simulink model "MotoSim"  (Simulink 8.9)
settings: Solver=ode1  StartTime=0.0  StopTime=Inf  FixedStep=0.01  RelTol=1e-3  EnableMultiTasking=on
PreLoadFcn:
  | clear all
  | close all
  | clc
  | 
  | currentFolder = pwd;
  | addpath(genpath(currentFolder));
values from neighbouring files (symbols this model uses):
  Stoptime = 60    [Initialize_Environment.m]    (also in Initialize_Environment_CDTS.m; Initialize_Environment_combined.m; Initialize_Sim.m)
undefined symbols (not defined in the file or in its folder): BATT_ELEC, BATT_OCV, BATT_THERMAL, EM, MC, soc0
libraries: simulink x4
settings Model: Creator=bring  LastModifiedBy=bring
settings OptimizationCC: ExpressionDepthLimit=2147483647
settings DebuggingCC: CheckSSInitialOutputMsg=off  SolverPrmCheckMsg=warning
settings SFSimCC: SimParseCustomCode=off
settings ConfigComp: CovSFcnEnable=off

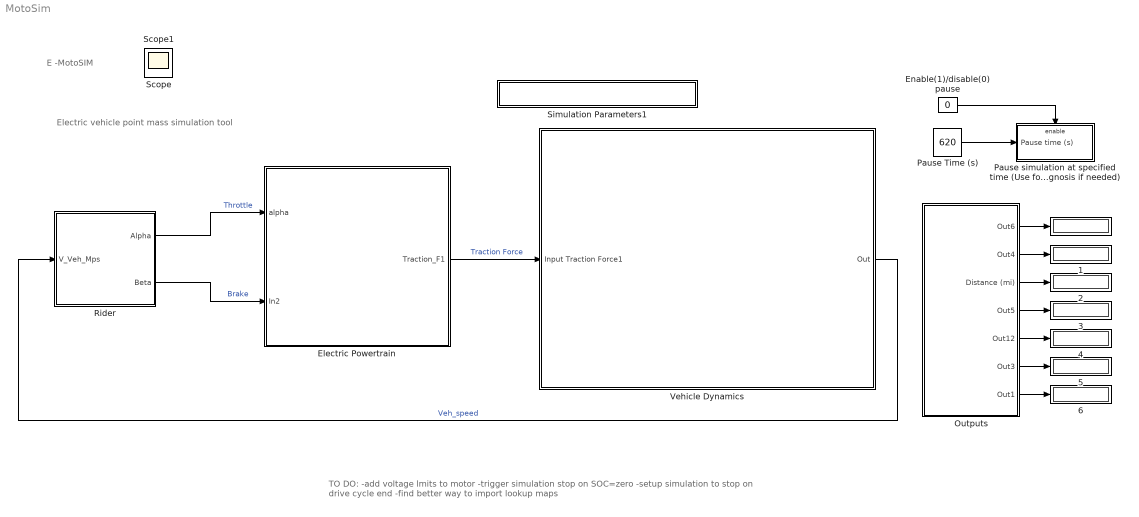
== system MotoSim ==
  note: TO DO:
      | -add voltage lmits to motor
      | -trigger simulation stop on SOC=zero
      | -setup simulation to stop on drive cycle end
      | -find better way to import lookup maps
  note: Electric vehicle point mass simulation tool
  note: E -MotoSIM
   {,1..6} (7 alike) : Display
  Electric Powertrain : Subsystem
      mask Display: image(imread('images/bike_powertrain.jpg'))
  Enable(1)/disable(0) pause : Constant  Value=0
  Outputs : Subsystem  mask(Outputs){}
  Pause Time (s) : Constant  Value=620
  Pause simulation at specified time (Use for diagnosis if needed) : Subsystem
  Rider : Subsystem  mask(Driver){kp=1, ki=0.1, kd=0.1}
      mask prompts: kp "Proportional Gain"; ki "Integral Gain"; kd "Derivative Gain"
      mask help: Please select the PID controller gains to improve the tracking response.
      mask Display: image(imread('Images/helmet.jpg'))
  Simulation Parameters1 : Subsystem  mask(Simulation Options){DRIV_Cycle=FUDS, VEH_Selection=sportbike_generic, M=250, TIRE_radius=0.3, CdA=0.38, maxBrakeTorque=2000, rowA=1.2, FrontSprocket_toothCt=23, RearSprocket_toothCt=54, regenPct=0, EM_MC_Selection=emrax268_PM150DZR, CELL_Selection=LiFePo4_generic, cellSeriesCount=134, cellParallelCount=1, cellCapacity=20, ENV_Selection=TRC_VDA, ambTemp=20, soc0=90, Grade_Value=0, Wind_Speed=0, iteration=1, DRIV_acc_flag=off, DRIV_acc_final_v=100}
      mask prompts: DRIV_Cycle "Driving Cycle"; VEH_Selection "Vehicle Selection"; M "Vehicle+Rider Mass (kg)"; TIRE_radius "Tire Radius"; maxBrakeTorque "Max Brake Torque"; rowA "Air Density"; FrontSprocket_toothCt "Fr Sprocket Teeth"; RearSprocket_toothCt "Rr Sprocket Teeth"; regenPct "Regen %"; EM_MC_Selection "Motor-MC Selection"; CELL_Selection "Battery Cell Selection"; cellSeriesCount "Series Cells"; cellParallelCount "Parallel Cells"; cellCapacity "Cell Capacity (Ah)"; ENV_Selection "Environment Selection"; ambTemp "Ambient Temperature (C)"; soc0 "Battey Initial SOC (%)"; Grade_Value "Road Grade Climb (degrees)"; Wind_Speed "Wind Speed (m/s)"; iteration "Driving Cycle Repetition"; DRIV_acc_flag "Acceleration Test"; DRIV_acc_final_v "Acceleration Test Final Velocity [kmph]"
      mask TypeOptions DRIV_Cycle: FHDS | FUDS | FUDS_fast | WLTP | US06 | US06_City_Cycle | US06_Highway_Cycle | Artemis_urban | Artemis_extra_urban | Artemis_highway | NEDC | PPIHC_CDTS
      mask TypeOptions VEH_Selection: sportbike_generic | EXR100 | RW-3x
      mask TypeOptions EM_MC_Selection: emrax268_PM150DZR | ME708_KDS48200e
      mask TypeOptions CELL_Selection: LiFePo4_generic | A123_ANR26650
      mask TypeOptions ENV_Selection: TRC_VDA | PikesPeak
      mask Display: text(.5,.5,'\fontsize{10}{\bfSimulation Settings}', 'hor','center','texmode','on');
  Vehicle Dynamics : Subsystem
      mask Display: image(imread('images/bike.jpg'))
  Scope : Scope
  Scope1 : Scope
  wires:
  Vehicle Dynamics/1(Out) -> Rider/1(V_Veh_Mps)  "Veh_speed"
  Rider/2(Beta) -> Electric Powertrain/2(In2)  "Brake"
  Rider/1(Alpha) -> Electric Powertrain/1(alpha)  "Throttle"
  Electric Powertrain/1(Traction_F1) -> Vehicle Dynamics/1(Input Traction Force1)  "Traction Force"
  Pause Time (s)/1 -> Pause simulation at specified time (Use for diagnosis if needed)/1(Pause time (s))
  Enable(1)/disable(0) pause/1 -> Pause simulation at specified time (Use for diagnosis if needed)/Enable
  Outputs/7(Out1) -> " 6"/1
  Outputs/6(Out3) -> " 5"/1
  Outputs/5(Out12) -> " 4"/1
  Outputs/4(Out5) -> " 3"/1
  Outputs/3(Distance (mi)) -> " 2"/1
  Outputs/2(Out4) -> " 1"/1
  Outputs/1(Out6) -> " "/1

== system MotoSim/Electric Powertrain ==
  alpha : Inport
  In2 : Inport  Port=2
  Battery Pack : Subsystem
      mask Display: image(imread('Images/pack.jpg'))
  Electric Motor  and  Motor Controller : Subsystem
      mask Display: image(imread('Images/idu.jpg'))
  Final Drive : Subsystem
      mask Display: image(imread('Images/gear.jpg'))
  Powertrain Controller : Subsystem
  Sum1 : Sum  Inputs=+|+
  Vehicle Brakes Front : Subsystem  mask(Brake){Brake_Position=[0 .14 0.31 0.46 0.76 1], Brake_Torque=[0 90.3 180.95 270.83 4600.4 6100]}
      mask prompts: Brake_Position "Brake Position"; Brake_Torque "Brake Torque"
      mask help:
      | This block calculates the brake torque using a 1D map between Brake position and Brake Torque
      | The inputs are the Brake Position array between 0 and 1 and the respective Brake Torque values.
      mask Display: image(imread('images/motoBrake.jpg'))
  Vehicle Brakes Rear : Subsystem  mask(Brake){Brake_Position=[0 .14 0.31 0.46 0.76 1], Brake_Torque=[0 90.3 180.95 270.83 4600.4 6100]}
      mask prompts: Brake_Position "Brake Position"; Brake_Torque "Brake Torque"
      mask help:
      | This block calculates the brake torque using a 1D map between Brake position and Brake Torque
      | The inputs are the Brake Position array between 0 and 1 and the respective Brake Torque values.
      mask Display: image(imread('images/motoBrake.jpg'))
  Vehicle Front Wheels : Subsystem
      mask Display: image(imread('Images/frTire_pirelli.jpg'))
  Vehicle Rear Wheels : Subsystem
      mask Display: image(imread('Images/rrTire_pirelli.jpg'))
  Traction_F1 : Outport
  wires:
  Vehicle Brakes Front/1(Out1) -> Vehicle Front Wheels/1(In1)
  alpha/1 -> Powertrain Controller/1(alpha)
  Vehicle Brakes Rear/1(Out1) -> Vehicle Rear Wheels/1(In1)
  In2/1 -> Powertrain Controller/2(In2)
  Powertrain Controller/3(Engine_Torque_Request) -> Vehicle Brakes Rear/2(Beta (Braking))
  Powertrain Controller/1(Engine_Torque_Request3) -> Vehicle Brakes Front/1(Beta (Braking))
  Electric Motor  and  Motor Controller/1(ICE_Speed) -> Final Drive/1(Torque EM)
  Final Drive/1(EM Torque) -> Vehicle Brakes Rear/1(Torque_out_REM_gearbox)
  Sum1/1 -> Traction_F1/1  "Traction Force"
  Vehicle Front Wheels/1(Out1) -> Sum1/1  "Front Traction Force"
  Vehicle Rear Wheels/1(Out1) -> Sum1/2  "Rear Traction Force"
  Powertrain Controller/2(Engine_Torque_Request4) -> Electric Motor  and  Motor Controller/1(Torque EM)

== system MotoSim/Outputs ==
  Battery Outputs : Subsystem
  Driver : Subsystem
  REM Outputs : Subsystem
  Vehicle Parameters : Subsystem
  Out6 : Outport
  Out4 : Outport  Port=2
  Distance (mi) : Outport  Port=3
  Out5 : Outport  Port=4
  Out12 : Outport  Port=5
  Out3 : Outport  Port=6
  Out1 : Outport  Port=7
  wires:
  Battery Outputs/3(Out2) -> Distance (mi)/1
  Battery Outputs/1(Out5) -> Out5/1
  REM Outputs/1(Out7) -> Out3/1
  REM Outputs/2(Out8) -> Out1/1
  Vehicle Parameters/1(Distance (mi)) -> Out4/1  "Distance (mi)"
  Vehicle Parameters/2(Out2) -> Out6/1
  Battery Outputs/2(Out1) -> Out12/1

== system MotoSim/Pause simulation at specified time (Use for diagnosis if needed) ==
  Pause time (s) : Inport
  Enable : EnablePort
  Add1 : Sum  Inputs=+-
  Assertion1 : Assertion  AssertionFailFcn=|  StopWhenAssertionFail=off
      | set_param(bdroot,'SimulationCommand','pause'),
      | disp(sprintf('\nSimulation paused.'))
  Clock1 : Clock
  Compare To Zero1 : simulink/Logic and Bit Operations/Compare To Zero  relop=~=  OutDataTypeStr=boolean
  wires:
  Clock1/1 -> Add1/1
  Compare To Zero1/1 -> Assertion1/1
  Add1/1 -> Compare To Zero1/1
  Pause time (s)/1 -> Add1/2

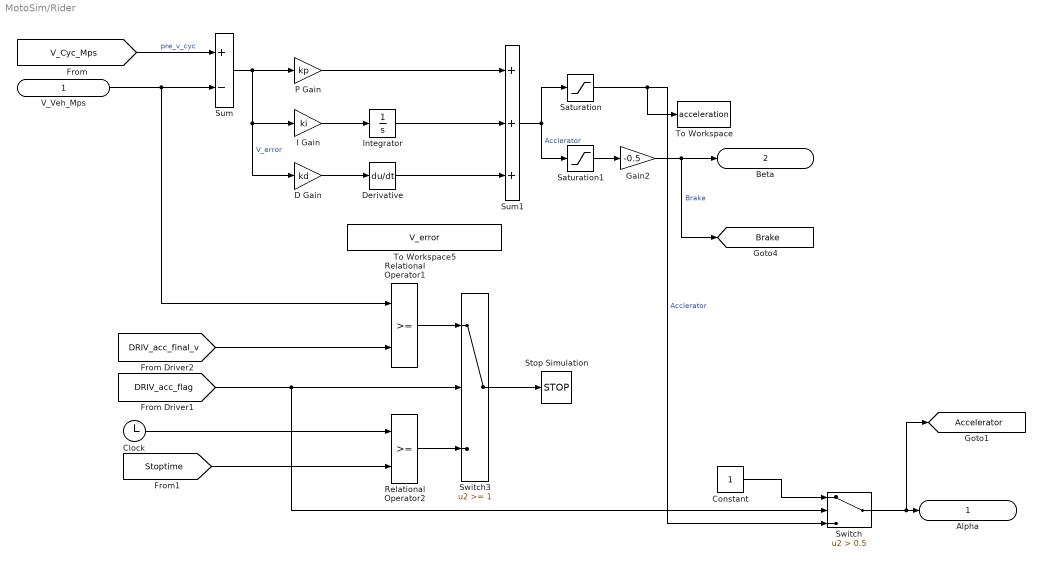
== system MotoSim/Rider ==
  V_Veh_Mps : Inport
  Clock : Clock
  Constant : Constant
  D Gain : Gain  Gain=kd
  Derivative : Derivative
  Gain2 : Gain  Gain=-0.5
  I Gain : Gain  Gain=ki
  Integrator : Integrator  UpperSaturationLimit=0.4
  P Gain : Gain  Gain=kp
  Relational Operator1 : RelationalOperator  RndMeth=Nearest  InputSameDT=on
  Relational Operator2 : RelationalOperator  RndMeth=Nearest  InputSameDT=on
  Saturation : Saturate  UpperLimit=1  LowerLimit=0
  Saturation1 : Saturate  UpperLimit=0  LowerLimit=-1
  Stop Simulation : Stop
  Sum : Sum  Inputs=+-
  Sum1 : Sum  Inputs=+++
  Switch : Switch  Criteria=u2 > Threshold  Threshold=0.5
  Switch3 : Switch  Threshold=1  SaturateOnIntegerOverflow=on  InputSameDT=on
  To Workspace : ToWorkspace  VariableName=acceleration  SampleTime=-1
  To Workspace5 : ToWorkspace  VariableName=V_error  SampleTime=-1
  Alpha : Outport
  Beta : Outport  Port=2
  tag scope: Accelerator=global, Brake=global
  wires:
  Gain2/1 -> [Brake], Beta/1  "Brake"
  Sum1/1 -> Saturation/1, Saturation1/1  "Acclerator"
  D Gain/1 -> Derivative/1
  I Gain/1 -> Integrator/1
  Saturation/1 -> To Workspace/1, Switch/3  "Acclerator"
  Saturation1/1 -> Gain2/1
  Clock/1 -> Relational Operator2/1
  [Stoptime] -> Relational Operator2/2
  [DRIV_acc_flag] -> Switch/2, Switch3/2
  Relational Operator1/1 -> Switch3/1
  [DRIV_acc_final_v] -> Relational Operator1/2
  Switch3/1 -> Stop Simulation/1
  Relational Operator2/1 -> Switch3/3
  Constant/1 -> Switch/1
  Switch/1 -> [Accelerator], Alpha/1
  Derivative/1 -> Sum1/3
  Integrator/1 -> Sum1/2
  P Gain/1 -> Sum1/1
  [V_Cyc_Mps] -> Sum/1  "pre_v_cyc"
  Sum/1 -> P Gain/1, D Gain/1, I Gain/1  "V_error"
  V_Veh_Mps/1 -> Relational Operator1/1, Sum/2

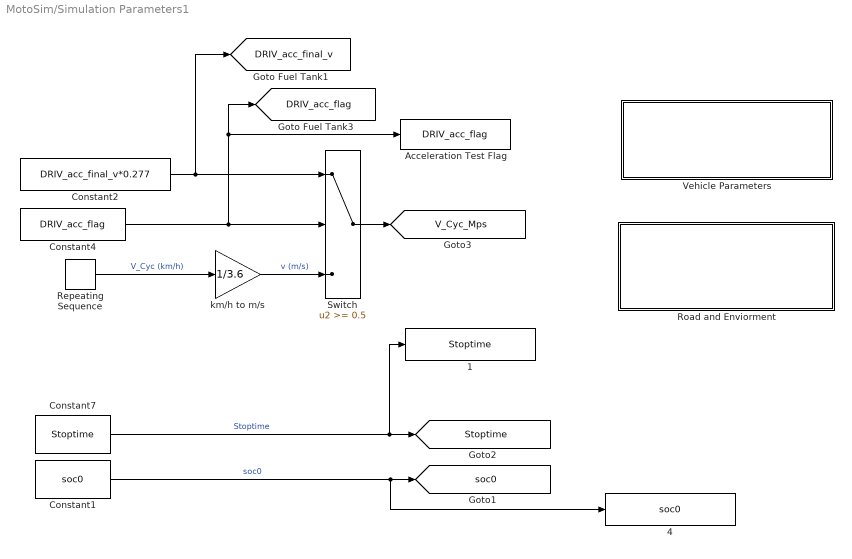
== system MotoSim/Simulation Parameters1 ==
  " 1" : ToWorkspace  VariableName=Stoptime  SampleTime=-1
      settings: MaxDataPoints=1
  " 4" : ToWorkspace  VariableName=soc0  SampleTime=-1
      settings: MaxDataPoints=1
  Acceleration Test Flag : ToWorkspace  VariableName=DRIV_acc_flag  SampleTime=-1
  Constant1 : Constant  Value=soc0
  Constant2 : Constant  Value=DRIV_acc_final_v*0.277
  Constant4 : Constant  Value=DRIV_acc_flag
  Constant7 : Constant  Value=Stoptime
  Repeating Sequence : simulink/Sources/Repeating Sequence  rep_seq_t=t_cyc  rep_seq_y=v_cyc
  Road and Enviorment : Subsystem
      mask Display: text(.5,.5,'\fontsize{10}{ Road and Environment}', 'hor','center','texmode','on');
  Switch : Switch  Threshold=0.5
  Vehicle Parameters : Subsystem
      mask Display: text(.5,.5,'\fontsize{10}{Vehicle Parameters}', 'hor','center','texmode','on');
  km/h to m/s : Gain  Gain=1/3.6
  tag scope: DRIV_acc_final_v=global, DRIV_acc_flag=global, Stoptime=global, V_Cyc_Mps=global, soc0=global
  wires:
  Switch/1 -> [V_Cyc_Mps]
  km/h to m/s/1 -> Switch/3  "v (m/s)"
  Constant2/1 -> Switch/1, [DRIV_acc_final_v]
  Constant4/1 -> Switch/2, [DRIV_acc_flag], Acceleration Test Flag/1
  Constant1/1 -> [soc0], " 4"/1  "soc0"
  Constant7/1 -> [Stoptime], " 1"/1  "Stoptime"
  Repeating Sequence/1 -> km/h to m/s/1  "V_Cyc (km/h)"

== system MotoSim/Vehicle Dynamics ==
  Input Traction Force1 : Inport
  Integrator1 : Integrator
  Saturation : Saturate  UpperLimit=inf  LowerLimit=0
  Vehicle Loads : Subsystem
  Vehicle_speed_Calculation : Subsystem
  Out : Outport
  tag scope: V_at_Wheel=global, Vehicle_Disctance_Travelled=global
  wires:
  Vehicle Loads/1(F (N)) -> Vehicle_speed_Calculation/2(In3)  "Vehicle_load (N)"
  Input Traction Force1/1 -> Vehicle_speed_Calculation/1(In1)
  Vehicle_speed_Calculation/1(Out1) -> Saturation/1  "Vehicle_Speed"
  Integrator1/1 -> [Vehicle_Disctance_Travelled]  "Vehicle_Distance"
  Saturation/1 -> Out/1, [V_at_Wheel], Integrator1/1  "Vehicle_Speed"

== system MotoSim/Electric Powertrain/Battery Pack ==
  Battery Parameters  Calculation : Subsystem
      mask Display:
      | color('blue');
      | fprintf('Battery Parameters Calculation')
  Battery to Cell : Subsystem
      mask Display:
      | color('blue');
      | fprintf('Battery to Cell')
  Cell : Subsystem
      mask Display:
      | color('blue');
      | fprintf('Cell: 1st Order Electrical Model')
  Cell to Batt : Subsystem
      mask Display:
      | color('blue');
      | fprintf('Cell to Battery')
  Current Limiter : Saturate  UpperLimit=180  LowerLimit=-60
  Divide : Product  Inputs=/*
  Memory : Memory
  Sum : Sum
  Thermal Dynamics : Subsystem
      mask Display:
      | color('blue');
      | fprintf('Thermal Dynamics')
  tag scope: P_from_Battery=global
  wires:
  Divide/1 -> Memory/1  "I_Batt_Req"
  Battery to Cell/1(Out1) -> Cell/1(In2)
  Cell/1(Out1) -> Cell to Batt/1(In1)
  Cell/2(Out2) -> Cell to Batt/2(In2)
  Cell to Batt/1(Out1) -> Divide/1
  Current Limiter/1 -> Battery Parameters  Calculation/1(current1), Battery to Cell/1(In1)  "I_Batt"
  Cell to Batt/2(Out3) -> [P_from_Battery]
  Memory/1 -> Current Limiter/1
  [P_Heat_Batt] -> Sum/1
  Sum/1 -> Divide/2  "P_Req"
  [P_Request_From_controller] -> Sum/2

== system MotoSim/Electric Powertrain/Electric Motor  and  Motor Controller ==
  Torque EM : Inport
  EM Max Torque Curve : Lookup  InputValues=EM.N_RPM  Table=EM.T_max_Peak  LookUpMeth=Interpolation-Use End Values  SaturateOnIntegerOverflow=on
  EM Min Torque Curve : Lookup  InputValues=EM.N_RPM  Table=EM.T_min_Peak  LookUpMeth=Interpolation-Use End Values  SaturateOnIntegerOverflow=on
  Power Request from Battery & Thermal : Subsystem
  Saturation Dynamic1 : simulink/Discontinuities/Saturation Dynamic  OutMin=[]  OutMax=[]  OutDataTypeStr=Inherit: Same as second input  OutDataType=sfix(16)  OutScaling=2^-10  DoSatur=off
  Transfer Fcn : TransferFcn  Denominator=[.1 1]
  ICE_Speed : Outport
  tag scope: T_From_REM=global, T_Max_Neg_From_REM=global, T_Max_Pos_From_REM=global
  wires:
  [REM_RPM] -> EM Max Torque Curve/1, EM Min Torque Curve/1, Power Request from Battery & Thermal/2(In1)  "REM_RPM"
  EM Max Torque Curve/1 -> Saturation Dynamic1/1, [T_Max_Pos_From_REM]
  EM Min Torque Curve/1 -> Saturation Dynamic1/3, [T_Max_Neg_From_REM]
  Torque EM/1 -> Transfer Fcn/1
  Saturation Dynamic1/1 -> ICE_Speed/1, [T_From_REM], Power Request from Battery & Thermal/1(In2)  "REM_torque"
  Transfer Fcn/1 -> Saturation Dynamic1/2

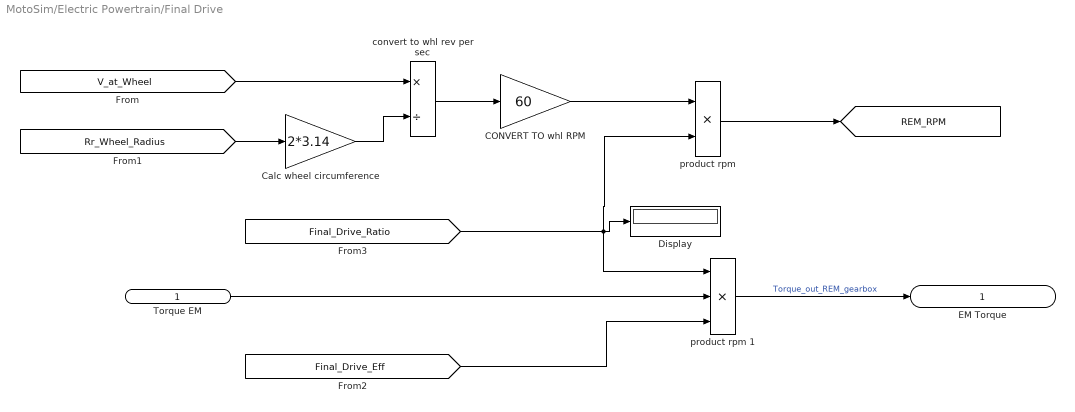
== system MotoSim/Electric Powertrain/Final Drive ==
  Torque EM : Inport
  "CONVERT TO whl RPM " : Gain  Gain=60
  Calc wheel circumference : Gain  Gain=2*3.14
  Display : Display
  "convert to whl rev per sec " : Product  Inputs=*/
  "product rpm " : Product  Inputs=**
  product rpm 1 : Product  Inputs=***
  EM Torque : Outport
  tag scope: REM_RPM=global
  wires:
  [V_at_Wheel] -> "convert to whl rev per sec "/1
  "convert to whl rev per sec "/1 -> "CONVERT TO whl RPM "/1
  product rpm 1/1 -> EM Torque/1  "Torque_out_REM_gearbox"
  [Rr_Wheel_Radius] -> Calc wheel circumference/1
  Calc wheel circumference/1 -> "convert to whl rev per sec "/2
  "CONVERT TO whl RPM "/1 -> "product rpm "/1
  "product rpm "/1 -> [REM_RPM]
  [Final_Drive_Ratio] -> Display/1, "product rpm "/2, product rpm 1/1
  [Final_Drive_Eff] -> product rpm 1/3
  Torque EM/1 -> product rpm 1/2

== system MotoSim/Electric Powertrain/Powertrain Controller ==
  alpha : Inport
  In2 : Inport  Port=2
  Braking Strategy : Subsystem
  Constant : Constant
  Constant1 : Constant  Value=4
  Memory2 : Memory
  Switch1 : Switch  Criteria=u2 > Threshold  Threshold=0.01
  Switch2 : Switch  Criteria=u2 > Threshold
  Traction Torque Strategy : Subsystem
  Engine_Torque_Request3 : Outport
  Engine_Torque_Request4 : Outport  Port=2
  Engine_Torque_Request : Outport  Port=3
  tag scope: Mode=global
  wires:
  Braking Strategy/2(Out2) -> Engine_Torque_Request/1
  In2/1 -> Braking Strategy/1(In1)
  Braking Strategy/3(Out3) -> Engine_Torque_Request3/1
  Switch1/1 -> Memory2/1  "REM_T_Request"
  alpha/1 -> Switch2/2, Switch1/2, Traction Torque Strategy/1(In1)
  Traction Torque Strategy/1(REM_Torque_Request) -> Switch1/1
  Braking Strategy/1(Out4) -> Switch1/3
  Memory2/1 -> Engine_Torque_Request4/1
  Switch2/1 -> [Mode]
  Constant/1 -> Switch2/1
  Constant1/1 -> Switch2/3

== system MotoSim/Electric Powertrain/Vehicle Brakes Front ==
  Beta (Braking) : Inport
  "ApplyNegForce " : Gain  Gain=-1
  Product : Product
  Out1 : Outport
  wires:
  Beta (Braking)/1 -> Product/1
  "ApplyNegForce "/1 -> Out1/1  "Net_Torque"
  Product/1 -> "ApplyNegForce "/1  "Net_Torque"
  [maxBrakeTorque] -> Product/2

== system MotoSim/Electric Powertrain/Vehicle Brakes Rear ==
  Torque_out_REM_gearbox : Inport
  Beta (Braking) : Inport  Port=2
  Product : Product
  Sum : Sum  Inputs=-+  SaturateOnIntegerOverflow=on  InputSameDT=on  OutDataTypeStr=Inherit: Same as first input
  Out1 : Outport
  wires:
  Torque_out_REM_gearbox/1 -> Sum/2  "Torque_out_REM_gearbox"
  Sum/1 -> Out1/1  "Rear_Net_Torque"
  Product/1 -> Sum/1
  Beta (Braking)/1 -> Product/1
  [maxBrakeTorque] -> Product/2

== system MotoSim/Electric Powertrain/Vehicle Front Wheels ==
  In1 : Inport
  Divide : Product  Inputs=*/
  Out1 : Outport
  wires:
  [Fr_Wheel_Radius] -> Divide/2
  In1/1 -> Divide/1
  Divide/1 -> Out1/1  "Tractive_Force_Front"

== system MotoSim/Electric Powertrain/Vehicle Rear Wheels ==
  In1 : Inport
  Divide : Product  Inputs=*/
  Out1 : Outport
  wires:
  [Rr_Wheel_Radius] -> Divide/2
  In1/1 -> Divide/1
  Divide/1 -> Out1/1  "Tractive_Force_Rear"

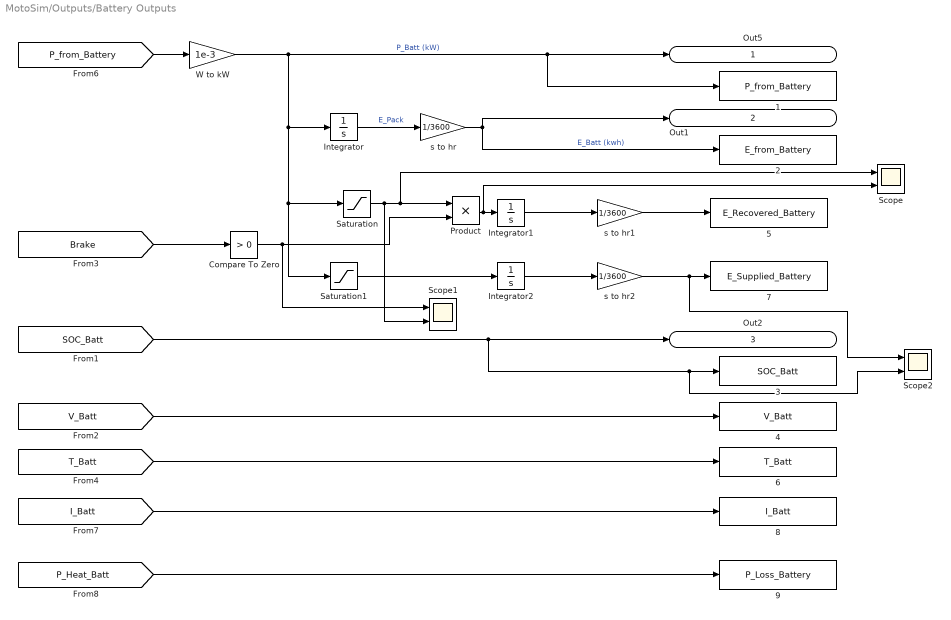
== system MotoSim/Outputs/Battery Outputs ==
  " 1" : ToWorkspace  VariableName=P_from_Battery  SampleTime=-1
  " 2" : ToWorkspace  VariableName=E_from_Battery  SampleTime=-1
  " 3" : ToWorkspace  VariableName=SOC_Batt  SampleTime=-1
  " 4" : ToWorkspace  VariableName=V_Batt  SampleTime=-1
  " 5" : ToWorkspace  VariableName=E_Recovered_Battery  SampleTime=-1
  " 6" : ToWorkspace  VariableName=T_Batt  SampleTime=-1
  " 7" : ToWorkspace  VariableName=E_Supplied_Battery  SampleTime=-1
  " 8" : ToWorkspace  VariableName=I_Batt  SampleTime=-1
  " 9" : ToWorkspace  VariableName=P_Loss_Battery  SampleTime=-1
  Compare To Zero : simulink/Logic and Bit Operations/Compare To Zero  relop=>  OutDataTypeStr=boolean
  Integrator : Integrator
  Integrator1 : Integrator
  Integrator2 : Integrator
  Product : Product  RndMeth=Zero
  Saturation : Saturate  UpperLimit=0  LowerLimit=-inf
  Saturation1 : Saturate  UpperLimit=inf  LowerLimit=0
  Scope : Scope  NumInputPorts=2
  Scope1 : Scope  NumInputPorts=2
  Scope2 : Scope  NumInputPorts=2
  W to kW : Gain  Gain=1e-3
  s to hr : Gain  Gain=1/3600
  s to hr1 : Gain  Gain=1/3600
  s to hr2 : Gain  Gain=1/3600
  Out5 : Outport
  Out1 : Outport  Port=2
  Out2 : Outport  Port=3
  wires:
  [P_from_Battery] -> W to kW/1
  Integrator/1 -> s to hr/1  "E_Pack"
  [SOC_Batt] -> Out2/1, Scope2/2, " 3"/1
  [V_Batt] -> " 4"/1
  [I_Batt] -> " 8"/1
  [P_Heat_Batt] -> " 9"/1
  s to hr/1 -> Out1/1, " 2"/1  "E_Batt (kwh)"
  s to hr1/1 -> " 5"/1
  Integrator1/1 -> s to hr1/1
  W to kW/1 -> Out5/1, " 1"/1, Integrator/1, Saturation1/1, Saturation/1  "P_Batt (kW)"
  s to hr2/1 -> Scope2/1, " 7"/1
  Integrator2/1 -> s to hr2/1
  Saturation1/1 -> Integrator2/1
  [Brake] -> Compare To Zero/1
  Product/1 -> Scope/2, Integrator1/1
  Saturation/1 -> Scope1/2, Scope/1, Product/1
  Compare To Zero/1 -> Scope1/1, Product/2
  [T_Batt] -> " 6"/1

== system MotoSim/Outputs/Driver ==
  To Workspace1 : ToWorkspace  VariableName=Brake_pedal  SampleTime=-1
  To Workspace6 : ToWorkspace  VariableName=Acc_pedal  SampleTime=-1
  wires:
  [Brake] -> To Workspace1/1
  [Accelerator] -> To Workspace6/1

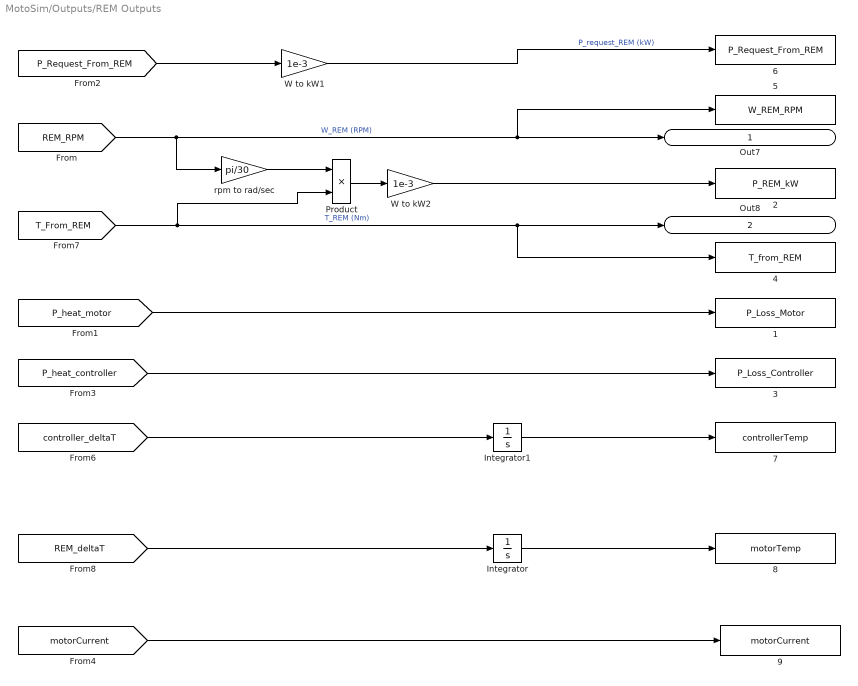
== system MotoSim/Outputs/REM Outputs ==
  " 1" : ToWorkspace  VariableName=P_Loss_Motor  SampleTime=-1
  " 2" : ToWorkspace  VariableName=P_REM_kW  SampleTime=-1
  " 3" : ToWorkspace  VariableName=P_Loss_Controller  SampleTime=-1
  " 4" : ToWorkspace  VariableName=T_from_REM  SampleTime=-1
  " 5" : ToWorkspace  VariableName=W_REM_RPM  SampleTime=-1
  " 6" : ToWorkspace  VariableName=P_Request_From_REM  SampleTime=-1
  " 7" : ToWorkspace  VariableName=controllerTemp  SampleTime=-1
  " 8" : ToWorkspace  VariableName=motorTemp  SampleTime=-1
  " 9" : ToWorkspace  VariableName=motorCurrent  SampleTime=-1
  Integrator : Integrator  InitialCondition=20
  Integrator1 : Integrator  InitialCondition=20
  Product : Product
  W to kW1 : Gain  Gain=1e-3
  W to kW2 : Gain  Gain=1e-3
  rpm to rad/sec : Gain  Gain=pi/30
  Out7 : Outport
  Out8 : Outport  Port=2
  wires:
  [T_From_REM] -> Product/2, " 4"/1, Out8/1  "T_REM (Nm)"
  [REM_RPM] -> " 5"/1, Out7/1, rpm to rad/sec/1  "W_REM (RPM)"
  W to kW1/1 -> " 6"/1  "P_request_REM (kW)"
  [P_Request_From_REM] -> W to kW1/1
  Product/1 -> W to kW2/1
  W to kW2/1 -> " 2"/1
  rpm to rad/sec/1 -> Product/1
  [P_heat_controller] -> " 3"/1
  [P_heat_motor] -> " 1"/1
  Integrator/1 -> " 8"/1
  Integrator1/1 -> " 7"/1
  [motorCurrent] -> " 9"/1
  [REM_deltaT] -> Integrator/1
  [controller_deltaT] -> Integrator1/1

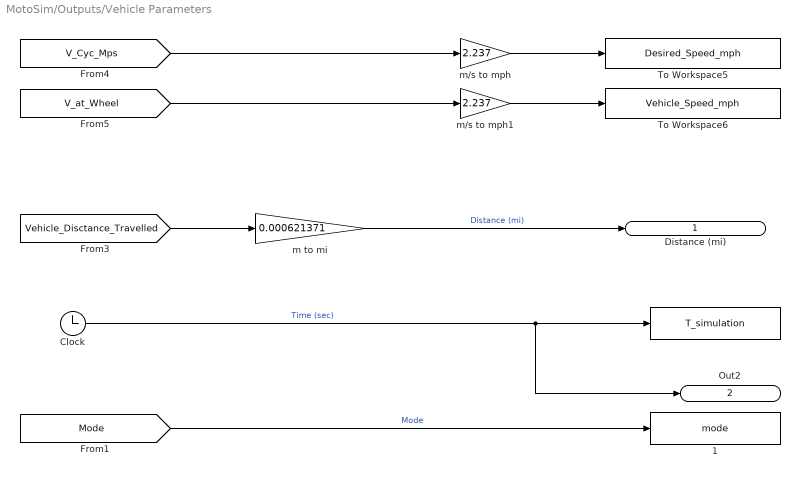
== system MotoSim/Outputs/Vehicle Parameters ==
  " " : ToWorkspace  VariableName=T_simulation  SampleTime=-1
  " 1" : ToWorkspace  VariableName=mode  SampleTime=-1
  Clock : Clock
  To Workspace5 : ToWorkspace  VariableName=Desired_Speed_mph  SampleTime=-1
  To Workspace6 : ToWorkspace  VariableName=Vehicle_Speed_mph  SampleTime=-1
  m to mi : Gain  Gain=0.000621371
  m/s to mph : Gain  Gain=2.237
  m/s to mph1 : Gain  Gain=2.237
  Distance (mi) : Outport
  Out2 : Outport  Port=2
  wires:
  [Vehicle_Disctance_Travelled] -> m to mi/1
  m to mi/1 -> Distance (mi)/1  "Distance (mi)"
  [V_Cyc_Mps] -> m/s to mph/1
  [V_at_Wheel] -> m/s to mph1/1
  m/s to mph/1 -> To Workspace5/1
  Clock/1 -> " "/1, Out2/1  "Time (sec)"
  m/s to mph1/1 -> To Workspace6/1
  [Mode] -> " 1"/1  "Mode"

== system MotoSim/Simulation Parameters1/Road and Enviorment ==
  Constant1 : Constant  Value=Wind_Speed
  Constant4 : Constant  Value=rowA
  Constant5 : Constant  Value=Grade_Value
  tag scope: Road_Grade=global, Row_Air=global, Wind_Speed=global
  wires:
  Constant4/1 -> [Row_Air]  "air density"
  Constant5/1 -> [Road_Grade]  "road grade"
  Constant1/1 -> [Wind_Speed]  "wind speed"

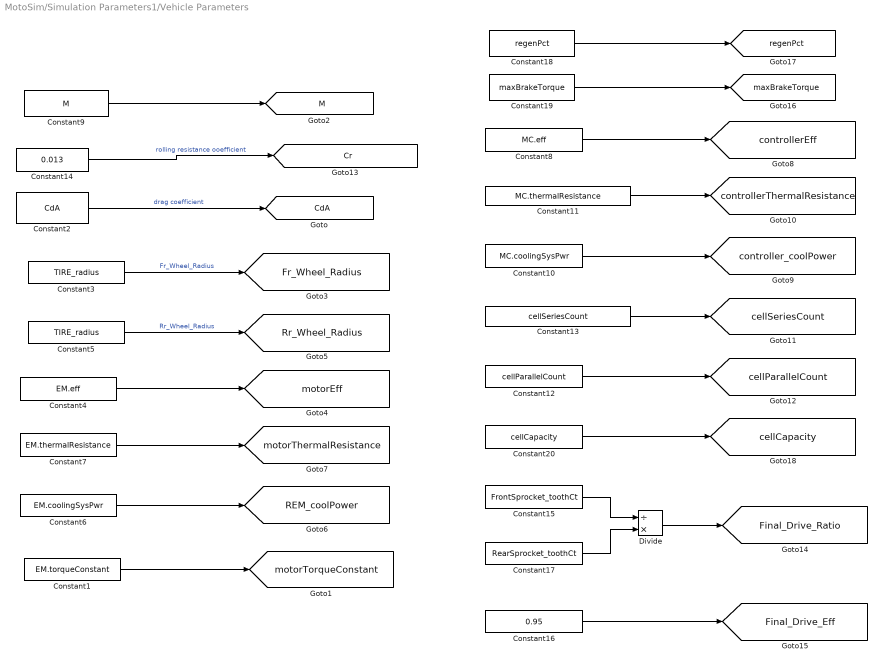
== system MotoSim/Simulation Parameters1/Vehicle Parameters ==
  Constant1 : Constant  Value=EM.torqueConstant
  Constant10 : Constant  Value=MC.coolingSysPwr
  Constant11 : Constant  Value=MC.thermalResistance
  Constant12 : Constant  Value=cellParallelCount
  Constant13 : Constant  Value=cellSeriesCount
  Constant14 : Constant  Value=0.013
  Constant15 : Constant  Value=FrontSprocket_toothCt
  Constant16 : Constant  Value=0.95
  Constant17 : Constant  Value=RearSprocket_toothCt
  Constant18 : Constant  Value=regenPct
  Constant19 : Constant  Value=maxBrakeTorque
  Constant2 : Constant  Value=CdA
  Constant20 : Constant  Value=cellCapacity
  Constant3 : Constant  Value=TIRE_radius
  Constant4 : Constant  Value=EM.eff
  Constant5 : Constant  Value=TIRE_radius
  Constant6 : Constant  Value=EM.coolingSysPwr
  Constant7 : Constant  Value=EM.thermalResistance
  Constant8 : Constant  Value=MC.eff
  Constant9 : Constant  Value=M
  Divide : Product  Inputs=/*
  tag scope: CdA=global, Cr=global, Final_Drive_Eff=global, Final_Drive_Ratio=global, Fr_Wheel_Radius=global, M=global, REM_coolPower=global, Rr_Wheel_Radius=global, cellCapacity=global, cellParallelCount=global, cellSeriesCount=global, controllerEff=global, controllerThermalResistance=global, controller_coolPower=global, maxBrakeTorque=global, motorEff=global, motorThermalResistance=global, motorTorqueConstant=global, regenPct=global
  wires:
  Constant2/1 -> [CdA]  "drag coefficient"
  Constant3/1 -> [Fr_Wheel_Radius]  "Fr_Wheel_Radius"
  Constant4/1 -> [motorEff]
  Constant5/1 -> [Rr_Wheel_Radius]  "Rr_Wheel_Radius"
  Constant7/1 -> [motorThermalResistance]
  Constant6/1 -> [REM_coolPower]
  Constant10/1 -> [controller_coolPower]
  Constant11/1 -> [controllerThermalResistance]
  Constant8/1 -> [controllerEff]
  Constant13/1 -> [cellSeriesCount]
  Constant12/1 -> [cellParallelCount]
  Constant14/1 -> [Cr]  "rolling resistance ooefficient"
  Constant1/1 -> [motorTorqueConstant]
  Constant16/1 -> [Final_Drive_Eff]
  Constant15/1 -> Divide/1
  Divide/1 -> [Final_Drive_Ratio]
  Constant17/1 -> Divide/2
  Constant19/1 -> [maxBrakeTorque]
  Constant18/1 -> [regenPct]
  Constant20/1 -> [cellCapacity]
  Constant9/1 -> [M]

== system MotoSim/Vehicle Dynamics/Vehicle Loads ==
  Aerodynamic  Drag : Subsystem
  Grade Force : Subsystem
  Roll Force : Subsystem
  Sum4 : Sum  Inputs=+++
  F (N) : Outport
  wires:
  Sum4/1 -> F (N)/1  "Road Load (N)"
  Roll Force/1(Power_roll) -> Sum4/3
  Aerodynamic  Drag/1(Drag Power) -> Sum4/2
  Grade Force/1(Drag Power) -> Sum4/1

== system MotoSim/Vehicle Dynamics/Vehicle_speed_Calculation ==
  In1 : Inport
  In3 : Inport  Port=2
  Divide : Product  Inputs=*//
  Integrator : Integrator  InitialCondition=0.0001  LimitOutput=on  LowerSaturationLimit=0
  Mass factor : Constant  Value=1.0
  Sum : Sum  Inputs=+-
  Out1 : Outport
  wires:
  Sum/1 -> Divide/1  "Net_Force"
  Divide/1 -> Integrator/1  "Vehicle_Acceleration"
  In1/1 -> Sum/1
  Integrator/1 -> Out1/1  "Vehicle_Speed"
  [M] -> Divide/2
  In3/1 -> Sum/2
  Mass factor/1 -> Divide/3

== system MotoSim/Electric Powertrain/Battery Pack/Battery Parameters  Calculation ==
  note: if I<0 --> CHARGE
  note: if I>0 --> DISCHARGE
  current1 : Inport
  Demux : Demux  Outputs=3
  OCV Calculation for Battery : Subsystem
      mask Display:
      | color('blue');
      | fprintf('OCV Calculation')
  "R0, C1, R1 Calculation for Battery" : Subsystem
      mask Display:
      | color('blue');
      | fprintf('R0, C1, R1, Calculation', 17)
  SOC Calculation for Battery : Subsystem
      mask Display:
      | color('blue');
      | fprintf('SOC Calculation')
  Switch CHARGE OR DISCHARGE : Switch  Criteria=u2 > Threshold
  tag scope: C1=global, R0=global, R1=global
  wires:
  Demux/3 -> [C1]
  Demux/2 -> [R1]
  Demux/1 -> [R0]
  Switch CHARGE OR DISCHARGE/1 -> Demux/1
  [BAT_Ch] -> Switch CHARGE OR DISCHARGE/3
  [BAT_DisCh] -> Switch CHARGE OR DISCHARGE/1
  current1/1 -> Switch CHARGE OR DISCHARGE/2, SOC Calculation for Battery/1(In1)

== system MotoSim/Electric Powertrain/Battery Pack/Battery to Cell ==
  In1 : Inport
  Divide : Product  Inputs=*/
  Out1 : Outport
  tag scope: I_Cell_Request=global
  wires:
  In1/1 -> Divide/1  "I_Bat_Req"
  [cellParallelCount] -> Divide/2
  Divide/1 -> [I_Cell_Request], Out1/1  "I_Cell_Req"

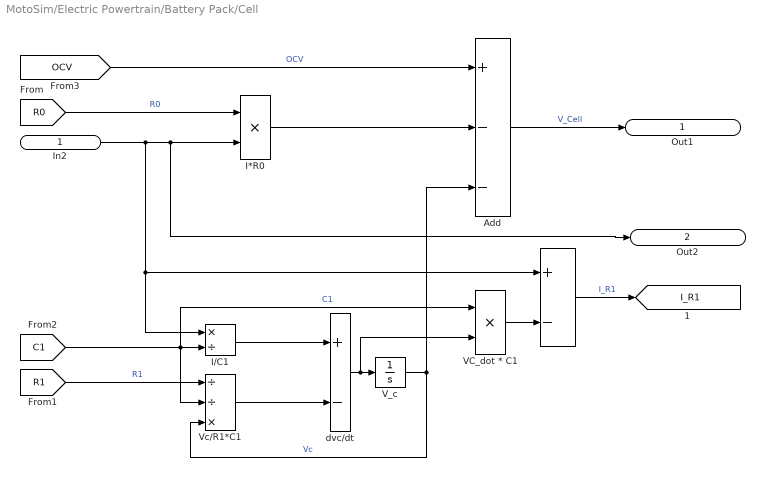
== system MotoSim/Electric Powertrain/Battery Pack/Cell ==
  In2 : Inport
  " " : Sum  Inputs=+-
  Add : Sum  Inputs=+--
  I*R0 : Product  RndMeth=Zero
  I/C1 : Product  Inputs=*/
  "VC_dot * C1 " : Product  RndMeth=Zero
  V_c : Integrator
  Vc/R1*C1 : Product  Inputs=//*
  dvc/dt : Sum  Inputs=+-
  Out1 : Outport
  Out2 : Outport  Port=2
  tag scope: I_R1=global
  wires:
  I*R0/1 -> Add/2
  [R0] -> I*R0/1  "R0"
  [OCV] -> Add/1  "OCV"
  In2/1 -> I/C1/1, " "/1, Out2/1, I*R0/2
  Add/1 -> Out1/1  "V_Cell"
  dvc/dt/1 -> "VC_dot * C1 "/2, V_c/1
  I/C1/1 -> dvc/dt/1
  [C1] -> I/C1/2, Vc/R1*C1/2, "VC_dot * C1 "/1  "C1"
  V_c/1 -> Vc/R1*C1/3, Add/3  "Vc"
  Vc/R1*C1/1 -> dvc/dt/2
  [R1] -> Vc/R1*C1/1  "R1"
  "VC_dot * C1 "/1 -> " "/2
  " "/1 -> [I_R1]  "I_R1"

== system MotoSim/Electric Powertrain/Battery Pack/Cell to Batt ==
  In1 : Inport
  In2 : Inport  Port=2
  multiply1 : Product  Inputs=**
  multiply2 : Product  Inputs=**
  multiply3 : Product  Inputs=**
  Out1 : Outport
  Out3 : Outport  Port=2
  tag scope: I_Batt=global, V_Batt=global
  wires:
  [cellSeriesCount] -> multiply1/1
  multiply1/1 -> [V_Batt], Out1/1, multiply3/1  "V_Batt"
  In1/1 -> multiply1/2
  In2/1 -> multiply2/1
  [cellParallelCount] -> multiply2/2
  multiply2/1 -> multiply3/2, [I_Batt]  "I_Batt"
  multiply3/1 -> Out3/1  "P_Batt"

== system MotoSim/Electric Powertrain/Battery Pack/Thermal Dynamics ==
  " 1" : Sum  Inputs=+-
  " 2" : Sum  Inputs=-+
  A : Constant  Value=BATT_THERMAL.A
  Integrator : Integrator  InitialCondition=20
  Pack Heat Generation : Subsystem
  Product : Product  Inputs=3  RndMeth=Zero
  Product1 : Product  RndMeth=Zero
  T_amb : Constant  Value=BATT_THERMAL.T_Amb
  h : Constant  Value=BATT_THERMAL.h
  m * c : Constant  Value=1/(BATT_THERMAL.m*BATT_THERMAL.c)
  tag scope: T_Batt=global
  wires:
  Pack Heat Generation/1(Out1) -> " 1"/1
  T_amb/1 -> " 2"/1
  Integrator/1 -> [T_Batt], " 2"/2  "T_Batt"
  Product/1 -> " 1"/2
  A/1 -> Product/2
  h/1 -> Product/1
  " 2"/1 -> Product/3
  " 1"/1 -> Product1/1
  m * c/1 -> Product1/2
  Product1/1 -> Integrator/1

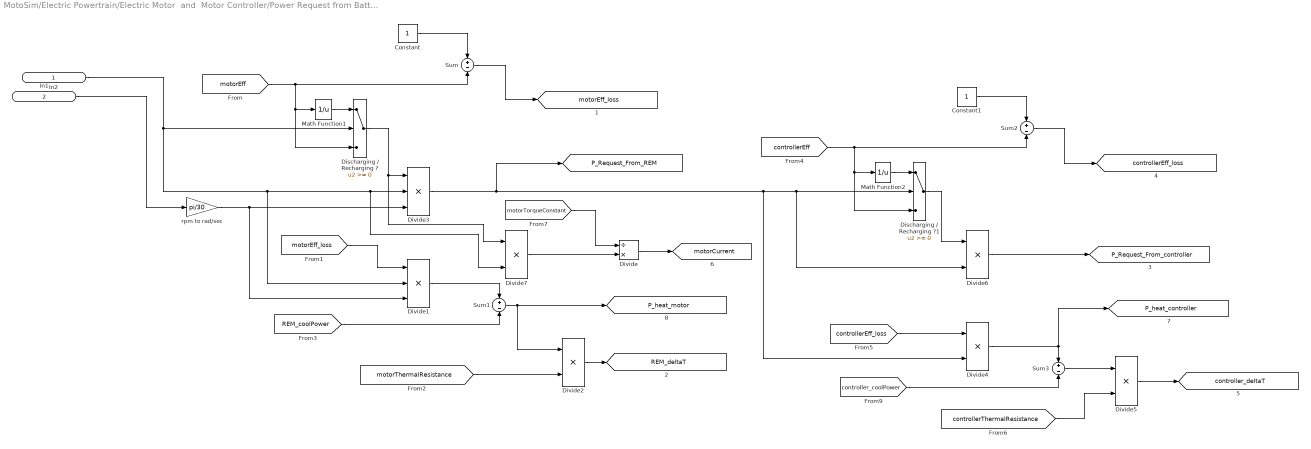
== system MotoSim/Electric Powertrain/Electric Motor  and  Motor Controller/Power Request from Battery & Thermal ==
  In2 : Inport
  In1 : Inport  Port=2
  Constant : Constant
  Constant1 : Constant
  Discharging / Recharging ? : Switch  SaturateOnIntegerOverflow=on  InputSameDT=on
  Discharging / Recharging ?1 : Switch  SaturateOnIntegerOverflow=on  InputSameDT=on
  Divide : Product  Inputs=/*
  Divide1 : Product  Inputs=***
  Divide{2,4..7} (5 alike) : Product  Inputs=**
  Divide3 : Product  Inputs=***
  Math Function1 : Math  Operator=reciprocal  SaturateOnIntegerOverflow=on
  Math Function2 : Math  Operator=reciprocal  SaturateOnIntegerOverflow=on
  Sum{,1..3} (4 alike) : Sum  Inputs=+-
  rpm to rad/sec : Gain  Gain=pi/30
  tag scope: P_Request_From_REM=global, P_Request_From_controller=global, P_heat_controller=global, P_heat_motor=global, REM_deltaT=global, controllerEff_loss=global, controller_deltaT=global, motorCurrent=global, motorEff_loss=global
  wires:
  In2/1 -> Discharging / Recharging ?/2, Divide1/2, Divide7/2, Divide3/2
  Discharging / Recharging ?/1 -> Divide7/1, Divide3/1
  In1/1 -> rpm to rad/sec/1
  [motorEff] -> Sum/2, Discharging / Recharging ?/3, Math Function1/1
  Math Function1/1 -> Discharging / Recharging ?/1
  rpm to rad/sec/1 -> Divide1/3, Divide3/3
  Sum/1 -> [motorEff_loss]
  Constant/1 -> Sum/1
  [motorEff_loss] -> Divide1/1
  Divide1/1 -> Sum1/1
  [REM_coolPower] -> Sum1/2
  Sum1/1 -> Divide2/1, [P_heat_motor]
  [motorThermalResistance] -> Divide2/2
  Divide2/1 -> [REM_deltaT]
  Divide5/1 -> [controller_deltaT]
  [controllerEff] -> Sum2/2, Discharging / Recharging ?1/3, Math Function2/1
  Constant1/1 -> Sum2/1
  Divide6/1 -> [P_Request_From_controller]
  [controllerThermalResistance] -> Divide5/2
  Divide4/1 -> [P_heat_controller], Sum3/1
  [controller_coolPower] -> Sum3/2
  Sum2/1 -> [controllerEff_loss]
  Math Function2/1 -> Discharging / Recharging ?1/1
  [controllerEff_loss] -> Divide4/1
  Sum3/1 -> Divide5/1
  Divide3/1 -> Divide4/2, Divide6/2, Discharging / Recharging ?1/2, [P_Request_From_REM]
  Discharging / Recharging ?1/1 -> Divide6/1
  Divide/1 -> [motorCurrent]
  [motorTorqueConstant] -> Divide/1
  Divide7/1 -> Divide/2

== system MotoSim/Electric Powertrain/Powertrain Controller/Braking Strategy ==
  In1 : Inport
  Abs1 : Abs
  Braking Strategy : Stateflow chart  TreatAsAtomicUnit=on
  Gain1 : Gain  Gain=-1
  Out4 : Outport
  Out2 : Outport  Port=2
  Out3 : Outport  Port=3
  wires:
  In1/1 -> Braking Strategy/1(Brake)
  Braking Strategy/2(Front_Wheels_Brake_Request) -> Out3/1  "Front_Wheels_Brake_Request"
  Braking Strategy/1(Rear_Wheels_Brake_Request) -> Out2/1  "Rear_Wheels_Brake_Request"
  [T_Max_Neg_From_REM] -> Abs1/1
  Abs1/1 -> Braking Strategy/3(T_Max_Neg_From_REM)
  Braking Strategy/3(REM_Brake_Torque_Request) -> Gain1/1
  Gain1/1 -> Out4/1  "REM_Brake_Torque_Request"
  [regenPct] -> Braking Strategy/2(data)

== system MotoSim/Electric Powertrain/Powertrain Controller/Traction Torque Strategy ==
  In1 : Inport
  Product : Product
  REM_Torque_Request : Outport
  wires:
  Product/1 -> REM_Torque_Request/1  "REM_Torque_Request"
  [T_Max_Pos_From_REM] -> Product/2
  In1/1 -> Product/1

== system MotoSim/Vehicle Dynamics/Vehicle Loads/Aerodynamic  Drag ==
  Constant : Constant  Value=0.5
  Drag force =1/2*row_a*Cd*Af*v2 : Product  Inputs=4  RndMeth=Zero
  Sum : Sum  Inputs=|++
  drag_v1 : Math  Operator=pow  SaturateOnIntegerOverflow=on
  square : Constant  Value=2
  Drag Power : Outport
  wires:
  square/1 -> drag_v1/2
  Constant/1 -> Drag force =1/2*row_a*Cd*Af*v2/1
  [CdA] -> Drag force =1/2*row_a*Cd*Af*v2/3
  [Row_Air] -> Drag force =1/2*row_a*Cd*Af*v2/2
  Drag force =1/2*row_a*Cd*Af*v2/1 -> Drag Power/1  "Drag_Force (N)"
  [V_at_Wheel] -> Sum/1
  Sum/1 -> drag_v1/1
  [Wind_Speed] -> Sum/2
  drag_v1/1 -> Drag force =1/2*row_a*Cd*Af*v2/4

== system MotoSim/Vehicle Dynamics/Vehicle Loads/Grade Force ==
  Fcn : Fcn  Expr=sin(u)
  Grade Force = M*g*sin(alpha) : Product  Inputs=3  RndMeth=Zero
  d to rad : Gain  Gain=pi/180
  gravity : Constant  Value=9.81
  Drag Power : Outport
  wires:
  Grade Force = M*g*sin(alpha)/1 -> Drag Power/1  "Grade_Force(N)"
  Fcn/1 -> Grade Force = M*g*sin(alpha)/3
  d to rad/1 -> Fcn/1
  [M] -> Grade Force = M*g*sin(alpha)/1
  gravity/1 -> Grade Force = M*g*sin(alpha)/2
  [Road_Grade] -> d to rad/1

== system MotoSim/Vehicle Dynamics/Vehicle Loads/Roll Force ==
  Display : Display
      settings: Decimation=5
  Display1 : Display
  Fcn : Fcn  Expr=cos(u)
  Fcn1 : Fcn  Expr=0.0048*(9/u(1))^0.5*(400/u(2))^0.25
  Mux : Mux  Inputs=2
  Roll_Force = Cr*M*g*cosd(road_grade) : Product  Inputs=4  RndMeth=Zero
  d to rad : Gain  Gain=pi/180
  "gravity accel (m/s^2) " : Constant  Value=9.81
  Power_roll : Outport
  wires:
  Roll_Force = Cr*M*g*cosd(road_grade)/1 -> Power_roll/1  "Roll_Force (N)"
  d to rad/1 -> Fcn/1
  Fcn/1 -> Roll_Force = Cr*M*g*cosd(road_grade)/4
  [Road_Grade] -> d to rad/1
  [M] -> Mux/2, Roll_Force = Cr*M*g*cosd(road_grade)/2
  Mux/1 -> Fcn1/1
  [Fr_Wheel_Radius] -> Mux/1
  Fcn1/1 -> Roll_Force = Cr*M*g*cosd(road_grade)/1, Display/1  "Cr"
  [Cr] -> Display1/1
  "gravity accel (m/s^2) "/1 -> Roll_Force = Cr*M*g*cosd(road_grade)/3

== system MotoSim/Electric Powertrain/Battery Pack/Battery Parameters  Calculation/OCV Calculation for Battery ==
  SoC vs. OCV : Lookup  InputValues=BATT_OCV.SoC  Table=BATT_OCV.OCV  LookUpMeth=Interpolation-Use End Values
  tag scope: OCV=global
  wires:
  [SOC_Batt] -> SoC vs. OCV/1
  SoC vs. OCV/1 -> [OCV]

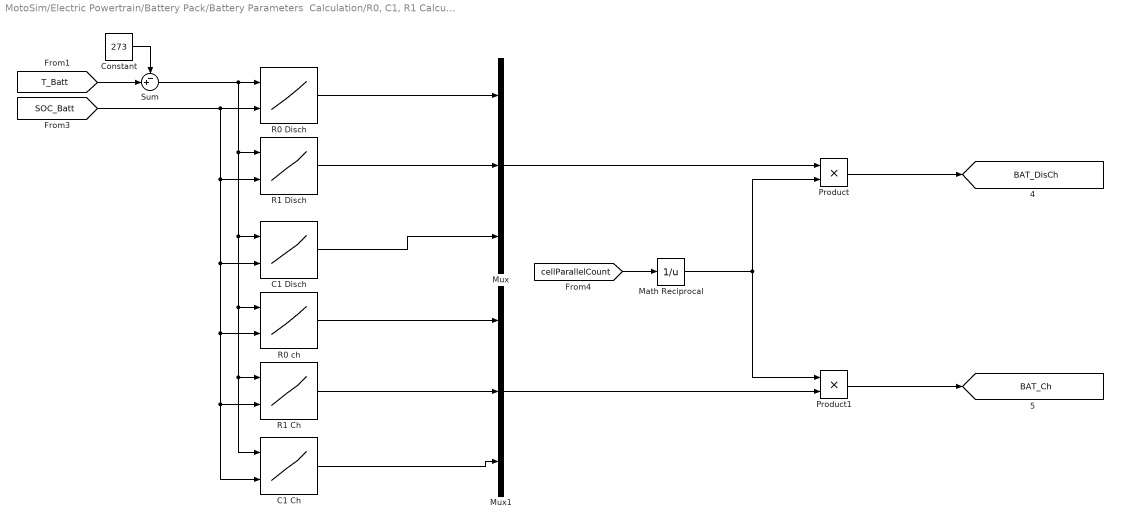
== system MotoSim/Electric Powertrain/Battery Pack/Battery Parameters  Calculation/R0, C1, R1 Calculation for Battery ==
  C1 Ch : Lookup2D  RowIndex=BATT_ELEC.temp_part  ColumnIndex=BATT_ELEC.soc_part  Table=BATT_ELEC.C1c  LookUpMeth=Interpolation-Use End Values
  C1 Disch : Lookup2D  RowIndex=BATT_ELEC.temp_part  ColumnIndex=BATT_ELEC.soc_part  Table=BATT_ELEC.C1d  LookUpMeth=Interpolation-Use End Values
  Constant : Constant  Value=273
  Math Reciprocal : Math  Operator=reciprocal  SaturateOnIntegerOverflow=on
  Mux : Mux  Inputs=3
  Mux1 : Mux  Inputs=3
  Product : Product
  Product1 : Product
  R0 Disch : Lookup2D  RowIndex=BATT_ELEC.temp_part  ColumnIndex=BATT_ELEC.soc_part  Table=BATT_ELEC.R0d  LookUpMeth=Interpolation-Use End Values
  R0 ch : Lookup2D  RowIndex=BATT_ELEC.temp_part  ColumnIndex=BATT_ELEC.soc_part  Table=BATT_ELEC.R0c  LookUpMeth=Interpolation-Use End Values
  R1 Ch : Lookup2D  RowIndex=BATT_ELEC.temp_part  ColumnIndex=BATT_ELEC.soc_part  Table=BATT_ELEC.R1c  LookUpMeth=Interpolation-Use End Values
  R1 Disch : Lookup2D  RowIndex=BATT_ELEC.temp_part  ColumnIndex=BATT_ELEC.soc_part  Table=BATT_ELEC.R1d  LookUpMeth=Interpolation-Use End Values
  Sum : Sum  Inputs=-+|
  tag scope: BAT_Ch=global, BAT_DisCh=global
  wires:
  Sum/1 -> C1 Ch/1, R1 Ch/1, R0 ch/1, C1 Disch/1, R1 Disch/1, R0 Disch/1
  [SOC_Batt] -> C1 Ch/2, R1 Ch/2, R0 ch/2, C1 Disch/2, R1 Disch/2, R0 Disch/2
  Mux1/1 -> Product1/2
  Constant/1 -> Sum/1
  [T_Batt] -> Sum/2
  R0 Disch/1 -> Mux/1
  C1 Disch/1 -> Mux/3
  R1 Disch/1 -> Mux/2
  R0 ch/1 -> Mux1/1
  R1 Ch/1 -> Mux1/2
  C1 Ch/1 -> Mux1/3
  Product/1 -> [BAT_DisCh]
  Mux/1 -> Product/1
  [cellParallelCount] -> Math Reciprocal/1
  Math Reciprocal/1 -> Product/2, Product1/1
  Product1/1 -> [BAT_Ch]

== system MotoSim/Electric Powertrain/Battery Pack/Battery Parameters  Calculation/SOC Calculation for Battery ==
  In1 : Inport
  Integrator : Integrator  InitialConditionSource=external  InitialCondition=soc0  LimitOutput=on  UpperSaturationLimit=100  LowerSaturationLimit=0
  Math Reciprocal : Math  Operator=reciprocal  SaturateOnIntegerOverflow=on
  Product1 : Product  Inputs=3  RndMeth=Zero
  Product2 : Product  RndMeth=Zero
  SoC % : Gain  Gain=100
  capacity : Constant  Value=-1/(3600)
  tag scope: SOC_Batt=global
  wires:
  Product1/1 -> SoC %/1
  capacity/1 -> Product1/1
  Math Reciprocal/1 -> Product1/3
  In1/1 -> Product1/2
  Integrator/1 -> [SOC_Batt]  "SoC_Batt"
  SoC %/1 -> Integrator/1
  [soc0] -> Integrator/2
  [cellCapacity] -> Product2/1
  [cellParallelCount] -> Product2/2
  Product2/1 -> Math Reciprocal/1

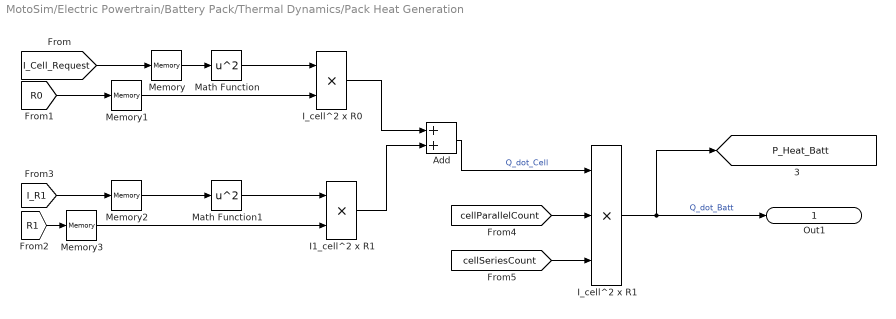
== system MotoSim/Electric Powertrain/Battery Pack/Thermal Dynamics/Pack Heat Generation ==
  Add : Sum
  I1_cell^2 x R1 : Product  RndMeth=Zero
  I_cell^2 x R0 : Product  RndMeth=Zero
  I_cell^2 x R1 : Product  Inputs=3  RndMeth=Zero
  Math Function : Math  Operator=square  SaturateOnIntegerOverflow=on
  Math Function1 : Math  Operator=square  SaturateOnIntegerOverflow=on
  Memory{,1..3} (4 alike) : Memory
  Out1 : Outport
  tag scope: P_Heat_Batt=global
  wires:
  [R0] -> Memory1/1
  [I_Cell_Request] -> Memory/1
  Math Function/1 -> I_cell^2 x R0/1
  [I_R1] -> Memory2/1
  [R1] -> Memory3/1
  I1_cell^2 x R1/1 -> Add/2
  I_cell^2 x R0/1 -> Add/1
  Add/1 -> I_cell^2 x R1/1  "Q_dot_Cell"
  I_cell^2 x R1/1 -> [P_Heat_Batt], Out1/1  "Q_dot_Batt"
  [cellParallelCount] -> I_cell^2 x R1/2
  [cellSeriesCount] -> I_cell^2 x R1/3
  Math Function1/1 -> I1_cell^2 x R1/1
  Memory/1 -> Math Function/1
  Memory1/1 -> I_cell^2 x R0/2
  Memory2/1 -> Math Function1/1
  Memory3/1 -> I1_cell^2 x R1/2

== stateflow chart Electric Powertrain/Powertrain Controller/Braking Strategy/Braking Strategy ==
  state No_Brake
    during:
    Front_Wheels_Brake_Request=0;
    Rear_Wheels_Brake_Request=0;
    REM_Brake_Torque_Request=0;
  state Normal_Brake
    during:
    Front_Wheels_Brake_Request=1*Brake;
    REM_Brake_Torque_Request=0*Brake*T_Max_Neg_From_REM;
    Rear_Wheels_Brake_Request=0*Brake;
  (default) -> No_Brake
  No_Brake -> Normal_Brake : [Brake>0.01]
  Normal_Brake -> No_Brake : [Brake<0.01]
  data: Brake input double; data input double; Rear_Wheels_Brake_Request output double; Front_Wheels_Brake_Request output double; T_Max_Neg_From_REM input double; REM_Brake_Torque_Request output double
